simulink model "BPSK"  (R2021a)
settings: Solver=VariableStepAuto  StartTime=0.0  StopTime=10.0  RelTol=1e-3
libraries: dsparch4 x1
settings Model: Creator=seman  LastModifiedBy=seman

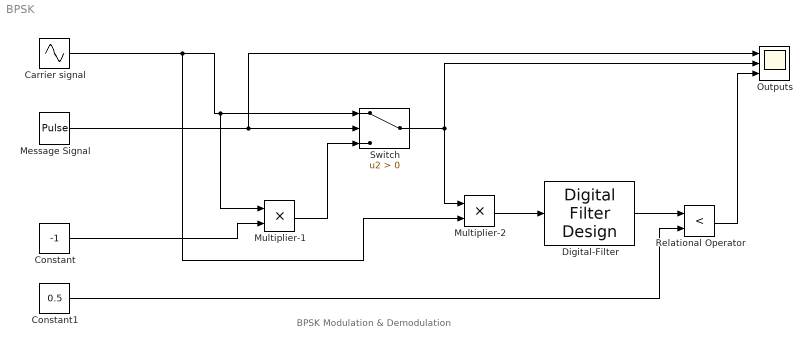
== system BPSK ==
  note: BPSK Modulation & Demodulation
  Carrier signal : Sin  Amplitude=2  Frequency=2*pi*4  SampleTime=0.01
  Constant : Constant  Value=-1
  Constant1 : Constant  Value=0.5
  "Digital-Filter " : dsparch4/Digital Filter Design  mwdsp_browser_bugfix_var=off
  Message Signal : DiscretePulseGenerator  PulseType=Time based  PulseWidth=50
  Multiplier-1 : Product
  Multiplier-2 : Product
  Outputs : Scope  NumInputPorts=3
  Relational Operator : RelationalOperator  Operator=<  OutDataTypeStr=boolean  RndMeth=Simplest
  Switch : Switch  Criteria=u2 > Threshold
  wires:
  Message Signal/1 -> Outputs/1, Switch/2
  Multiplier-1/1 -> Switch/3
  Constant/1 -> Multiplier-1/2
  Switch/1 -> Multiplier-2/1, Outputs/2
  Multiplier-2/1 -> "Digital-Filter "/1
  Carrier signal/1 -> Multiplier-2/2, Multiplier-1/1, Switch/1
  "Digital-Filter "/1 -> Relational Operator/1
  Constant1/1 -> Relational Operator/2
  Relational Operator/1 -> Outputs/3
